simulink subsystem "rss_RefCurrCalc"  (R2023a)
settings: Solver=VariableStepAuto  StartTime=0.0  StopTime=5  RelTol=1e-3
undefined symbols (not defined in the file): Cdbl_iPhCurrPeakVal, Cdbl_numPPNumMinVal, Cdbl_psiPermMagFlxMaxVal, Cdbl_psiPermMagFlxMinVal, Cdbl_psiPermMagFlxPeakVal, Cdbl_trqTqMaxVal, Cdbl_trqTqPeakVal
libraries: lib_conversion x5, lib_configurable_parameter x1
settings Model: DefaultTestHarness=rss_ReferenceCurrentGenerator_thu  Creator=CAV2OFO  LastModifiedBy=xiaoqiang.yuan
settings OptimizationCC: ReuseModelBlockBuffer=off

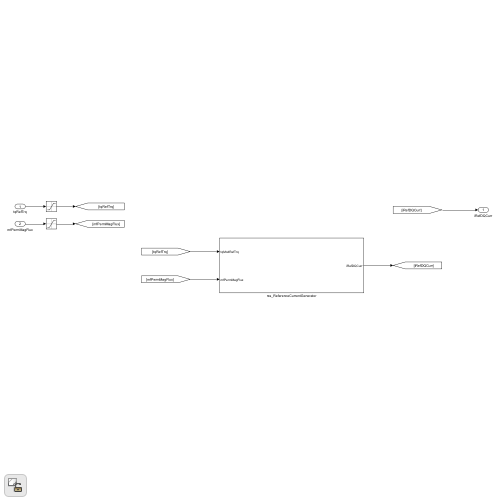
[thumbnail: Simulink's stored preview of the top-level diagram]
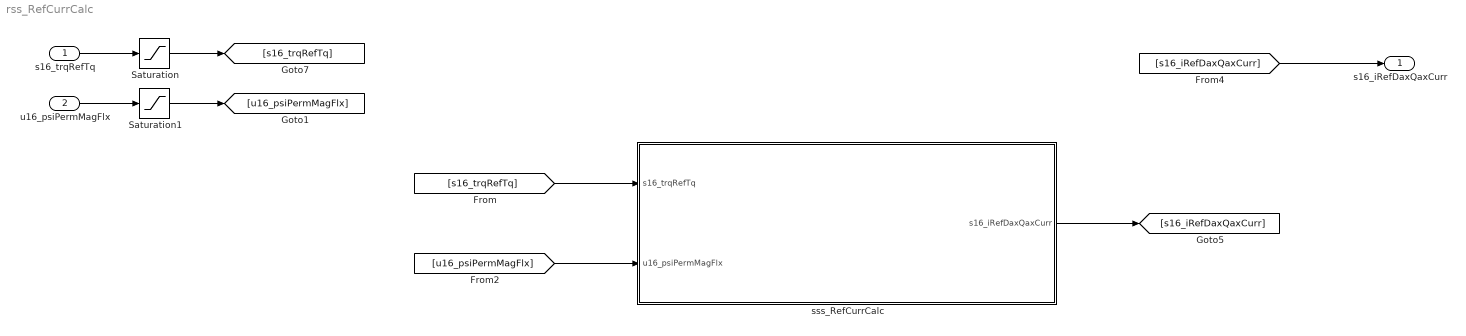
== system rss_RefCurrCalc ==
  s16_trqRefTq : Inport  OutDataTypeStr=dt_Standardize_s16p15b0
  u16_psiPermMagFlx : Inport  Port=2  OutDataTypeStr=dt_Standardize_u16p15b0
  Saturation : Saturate  UpperLimit=Cdbl_trqTqMaxVal  LowerLimit=-Cdbl_trqTqMaxVal
  Saturation1 : Saturate  UpperLimit=Cdbl_psiPermMagFlxMaxVal  LowerLimit=Cdbl_psiPermMagFlxMinVal
  sss_RefCurrCalc : Subsystem
  s16_iRefDaxQaxCurr : Outport  OutDataTypeStr=dt_Standardize_s16p15b0
  wires:
  s16_trqRefTq/1 -> Saturation/1
  Saturation1/1 -> [u16_psiPermMagFlx]
  Saturation/1 -> [s16_trqRefTq]
  [s16_iRefDaxQaxCurr] -> s16_iRefDaxQaxCurr/1
  [s16_trqRefTq] -> sss_RefCurrCalc/1(s16_trqRefTq)
  [u16_psiPermMagFlx] -> sss_RefCurrCalc/2(u16_psiPermMagFlx)
  sss_RefCurrCalc/1(s16_iRefDaxQaxCurr) -> [s16_iRefDaxQaxCurr]
  u16_psiPermMagFlx/1 -> Saturation1/1

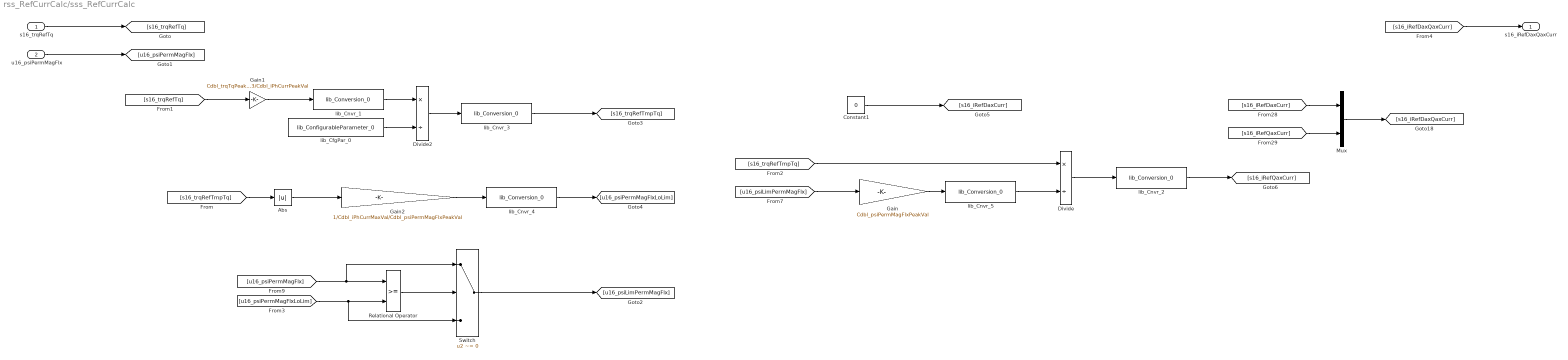
== system rss_RefCurrCalc/sss_RefCurrCalc ==
  s16_trqRefTq : Inport
  u16_psiPermMagFlx : Inport  Port=2
  Abs : Abs  SaturateOnIntegerOverflow=off
  Constant1 : Constant  Value=0  OutDataTypeStr=dt_Standardize_s16p15b0
  Divide : Product  Inputs=*/  OutDataTypeStr=Inherit: Inherit via back propagation  RndMeth=Simplest
  Divide2 : Product  Inputs=*/  OutDataTypeStr=Inherit: Inherit via back propagation  RndMeth=Simplest
  Gain : Gain  Gain=Cdbl_psiPermMagFlxPeakVal  OutDataTypeStr=Inherit: Inherit via back propagation
  Gain1 : Gain  Gain=Cdbl_trqTqPeakVal*2/3/Cdbl_iPhCurrPeakVal  OutDataTypeStr=Inherit: Inherit via back propagation
  Gain2 : Gain  Gain=1/Cdbl_iPhCurrMaxVal/Cdbl_psiPermMagFlxPeakVal  OutDataTypeStr=Inherit: Inherit via back propagation
  Mux : Mux  Inputs=2
  Relational Operator : RelationalOperator  OutDataTypeStr=boolean  RndMeth=Simplest  InputSameDT=off
  Switch : Switch  Criteria=u2 ~= 0  SaturateOnIntegerOverflow=off  InputSameDT=off
  lib_CfgPar_0 : lib_configurable_parameter/lib_ConfigurableParameter_0  lb_parCnfgPar=Gu8_numPPNum_C  lb_parDataType=Inherit: Inherit from 'Constant value'  lb_parUpLim=Cdbl_numPPNumMaxVal  lb_parLowLim=Cdbl_numPPNumMinVal
  lib_Cnvr_1 : lib_conversion/lib_Conversion_0  lb_parDataType=fixdt(1,16)  lb_parOutpMaxVal=Cdbl_trqTqMaxVal*Cdbl_trqTqPeakVal*2/3/Cdbl_iPhCurrPeakVal  lb_parOutpMinVal=[]  RndMeth=Simplest  lb_parSatFlag=off
  lib_Cnvr_2 : lib_conversion/lib_Conversion_0  lb_parDataType=dt_Standardize_s16p15b0  lb_parOutpMaxVal=[]  lb_parOutpMinVal=[]  RndMeth=Simplest  lb_parSatFlag=off
  lib_Cnvr_3 : lib_conversion/lib_Conversion_0  lb_parDataType=fixdt(1,16)  lb_parOutpMaxVal=Cdbl_trqTqMaxVal*Cdbl_trqTqPeakVal*2/3/double(Cdbl_numPPNumMinVal)/Cdbl_iPhCurrPeakVal  lb_parOutpMinVal=[]  RndMeth=Simplest  lb_parSatFlag=off
  lib_Cnvr_4 : lib_conversion/lib_Conversion_0  lb_parDataType=dt_Standardize_u16p15b0  lb_parOutpMaxVal=[]  lb_parOutpMinVal=[]  RndMeth=Simplest  lb_parSatFlag=off
  lib_Cnvr_5 : lib_conversion/lib_Conversion_0  lb_parDataType=fixdt(0,16)  lb_parOutpMaxVal=Cdbl_psiPermMagFlxPeakVal  lb_parOutpMinVal=[]  RndMeth=Simplest  lb_parSatFlag=off
  s16_iRefDaxQaxCurr : Outport
  wires:
  [u16_psiLimPermMagFlx] -> Gain/1
  lib_Cnvr_5/1 -> Divide/2
  Gain/1 -> lib_Cnvr_5/1
  lib_Cnvr_1/1 -> Divide2/1
  [s16_iRefDaxQaxCurr] -> s16_iRefDaxQaxCurr/1
  [s16_iRefDaxCurr] -> Mux/1
  [s16_iRefQaxCurr] -> Mux/2
  Mux/1 -> [s16_iRefDaxQaxCurr]
  Abs/1 -> Gain2/1
  lib_Cnvr_4/1 -> [u16_psiPermMagFlxLoLim]
  [s16_trqRefTq] -> Gain1/1
  Gain2/1 -> lib_Cnvr_4/1
  [s16_trqRefTmpTq] -> Abs/1
  [s16_trqRefTmpTq] -> Divide/1
  [u16_psiPermMagFlx] -> Switch/1, Relational Operator/1
  Divide/1 -> lib_Cnvr_2/1
  Divide2/1 -> lib_Cnvr_3/1
  Gain1/1 -> lib_Cnvr_1/1
  lib_CfgPar_0/1 -> Divide2/2
  lib_Cnvr_2/1 -> [s16_iRefQaxCurr]
  s16_trqRefTq/1 -> [s16_trqRefTq]
  Switch/1 -> [u16_psiLimPermMagFlx]
  lib_Cnvr_3/1 -> [s16_trqRefTmpTq]
  u16_psiPermMagFlx/1 -> [u16_psiPermMagFlx]
  Constant1/1 -> [s16_iRefDaxCurr]
  Relational Operator/1 -> Switch/2
  [u16_psiPermMagFlxLoLim] -> Switch/3, Relational Operator/2
